simulink model "ImpedanceControl"  (R2017a)
settings: Solver=ode23t  StartTime=0.0  StopTime=10.0  RelTol=1e-1
values from neighbouring files (symbols this model uses):
  Kd = 500*eye(6)    [Initial.m]
  Kp = 2500*eye(6)    [Initial.m]
  Md = 100*eye(6)    [Initial.m]
  Md_inv = inv(Md)    [Initial.m]
libraries: mblibv1 x72
(part 4 of 14)

== matlab function ImpedanceControl/Impedance Control/JA_dot*qdot ==
  data: q input; res output; dq input
function res  = JA_dot(q,dq)
%JA_DOT
%    JA_DOT = JA_DOT(DQ1,DQ2,DQ3,DQ4,DQ5,DQ6,Q1,Q2,Q3,Q4,Q5,Q6)

%    This function was generated by the Symbolic Math Toolbox version 7.2.
%    01-May-2017 19:37:21
dq1=dq(1);
dq2=dq(2);
dq3=dq(3);
dq4=dq(4);
dq5=dq(5);
dq6=dq(6);
q1=q(1);
q2=q(2);
q3=q(3);
q4=q(4);
q5=q(5);
q6=q(6);
